simulink subsystem "PieroCPModelZ"  (R2023b)
settings: Solver=VariableStepAuto  StartTime=0.0  StopTime=10.0  RelTol=1e-3
settings Model: Creator=Carlos  LastModifiedBy=Carlos

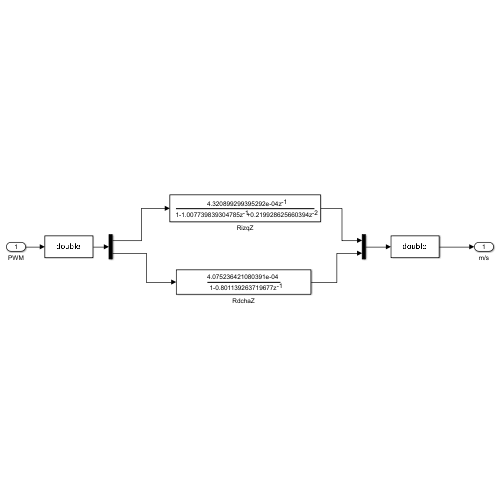
[thumbnail: Simulink's stored preview of the top-level diagram]
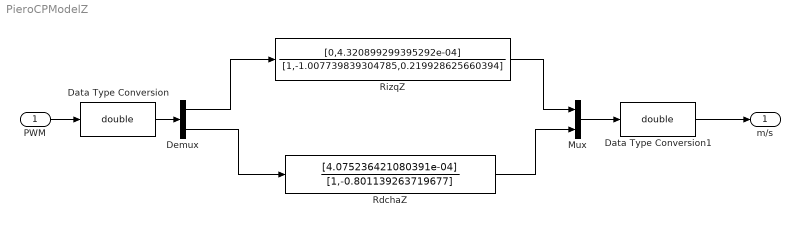
== system PieroCPModelZ ==
  PWM : Inport
  Data Type Conversion : DataTypeConversion  OutDataTypeStr=double  SaturateOnIntegerOverflow=off  RndMeth=Floor
  Data Type Conversion1 : DataTypeConversion  OutDataTypeStr=double  SaturateOnIntegerOverflow=off  RndMeth=Floor
  Demux : Demux  Outputs=2
  Mux : Mux  Inputs=2
  RdchaZ : DiscreteFilter  Numerator=[4.075236421080391e-04]  Denominator=[1,-0.801139263719677]
  RizqZ : DiscreteFilter  Numerator=[0,4.320899299395292e-04]  Denominator=[1,-1.007739839304785,0.219928625660394]
  m/s : Outport
  wires:
  Demux/1 -> RizqZ/1
  Demux/2 -> RdchaZ/1
  RizqZ/1 -> Mux/1
  RdchaZ/1 -> Mux/2
  PWM/1 -> Data Type Conversion/1
  Mux/1 -> Data Type Conversion1/1
  Data Type Conversion/1 -> Demux/1
  Data Type Conversion1/1 -> m/s/1
